simulink model "vfs_unity"  (R2022a)
settings: Solver=FixedStepAuto  StartTime=0.0  StopTime=inf  FixedStep=0.02  RelTol=1e-3
undefined symbols (not defined in the file): alpha, Angular, gd, Kc, Linear, ros_freq, Rx, Ry, Rz, T, var_max, X, Y, Z
libraries: simlib_vpc_coremath x35, robotlib x26, simlib_vpc_basic x14, simlib_vpc_gp x7, dspmtrx3 x5
(part 2 of 2)

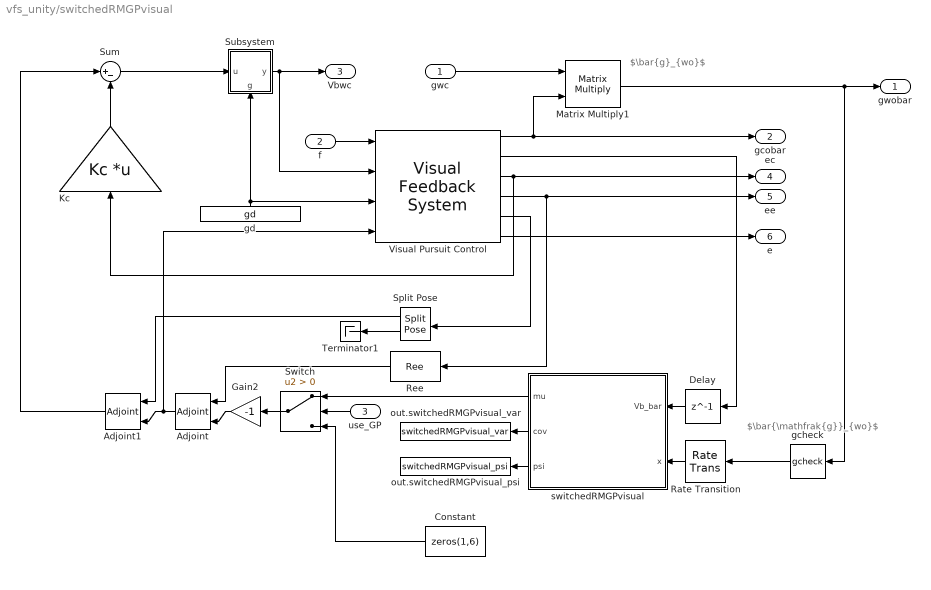
== system vfs_unity/switchedRMGPvisual ==
  note: $\bar{g}_{wo}$
  note: $\bar{\mathfrak{g}}_{wo}$
  gwc : Inport
  f : Inport  Port=2
  use_GP : Inport  Port=3
  Adjoint : simlib_vpc_basic/Adjoint  adjointtype=orientation
      settings: SourceProductName=VPC Library
  Adjoint1 : simlib_vpc_basic/Adjoint  adjointtype=orientation
      settings: SourceProductName=VPC Library
  Constant : Constant  Value=zeros(1,6)
  Delay : Delay  DelayLength=1
  Gain2 : Gain  Gain=-1
  Kc : Gain  Gain=Kc  Multiplication=Matrix(K*u) (u vector)
  Matrix Multiply1 : Product  Multiplication=Matrix(*)
  Rate Transition : RateTransition
  Ree : simlib_vpc_coremath/Ree
      settings: SourceProductName=VPC Library
  Split Pose : simlib_vpc_coremath/Split Pose  show_R=on  show_p=on
      settings: SourceProductName=VPC Library
  Subsystem : Subsystem
      settings: PortSchema="{\"entries\":[{\"content\":{\"sides\":[{\"content\":{\"connectorIds\":[\"In1\"]},\"type\":\"ConnectorPlacement.EquallySpacedRectSide\",\"uuid\":\"72e68008-5c4a-43a9-a560-64c6a31a0c08\"},{\"content\":{\"connectorIds\":[\"Out1\"],\"side\":\"RIGHT\"},\"type\":\"ConnectorPlacement.EquallySpacedRectSide\",\"uuid\":\"da07f5ff-2b2c-4c55-a2f2-34e133777503\"},{\"content\":{\"connectorIds\":[],\"side\":\"TOP\"},\"type\":\"ConnectorPlacement.EquallySpacedRectSide\",\"uuid\":\"6d174428-4364-4e89-aba7-4e9864808ab5\"},{\"content\":{\"connectorIds\":[\"In2\"],\"side\":\"BOTTOM\"},\"type\":\"ConnectorPlacement.EquallySpacedRectSide\",\"uuid\":\"f9633104-9c11-4d21-90a7-e0f886d9e92d\"},{\"content\":{\"connectorIds\":[],\"side\":\"HIDDEN\"},\"type\":\"ConnectorPlacement.EquallySpacedRectSide\",\"uuid\":\"662f08ae-9279-4a4f-85ea-81d97ead27d9\"}]},\"type\":\"ConnectorPlacement.EquallySpacedConnector\",\"uuid\":\"f3cd156c-cccd-47c6-b81c-6113f78efd58\"}],\"packageUris\":[\"http://schema.mathworks.com/mf0/Connector/R2020b\"],\"version\":\"1.0\"}"
      mask Display:
      | % Glitch in Matlab: If you define a line whose starting point and end point
      | % is equal, then the entire mask block is plotted in bold
      | plot([0,0],[0,0])
      | 
      | % Draw box
      | indent = 0.3;
      | ang=[0:0.2:pi/2, pi/2];
      | plot([0,1-indent],[0,0])
      | xp=indent*sin(ang)+1-indent;
      | yp=indent-indent*cos(ang);
      | plot(xp,yp);
      | plot([1,1,indent],[indent,1,1])
      | xp=indent-indent*sin(ang);
      | yp=1-indent+indent*cos(ang);
      | plot(xp,yp);
      | plot([0,0],[1-indent,0])
      | 
      | % Write label & ports
      | disp('-Ad_{(g_d)}','texmode','on')
      | text(0.5,0.2,'\fontsize{7}g_d','texmode','on')
  Sum : Sum  Inputs=|+-
  Switch : Switch  Criteria=u2 > Threshold  SaturateOnIntegerOverflow=off  InputSameDT=off
  Terminator1 : Terminator
  Visual Pursuit Control : simlib_vpc_basic/Visual Feedback System  gd_source=external  gd_value=[eye(4,3),ones(4,1)]  gcobar0=gco_init  Ke_source=internal  Ke=Ke  projection=on  camtype=Pinhole  fo=fp  lambda=lambda  show_Vbwo=on  show_ec=on  show_gce=on  show_ee=on  show_gee=off  show_e=on  show_nu=off  show_dgcobar=off  show_ue_aux=on
      settings: SourceProductName=VPC Library
  gcheck : simlib_vpc_coremath/gcheck
      settings: SourceProductName=VPC Library
  gd : Constant  Value=gd
  out.switchedRMGPvisual_psi : ToWorkspace  VariableName=switchedRMGPvisual_psi  SaveFormat=Structure With Time  SampleTime=-1
  out.switchedRMGPvisual_var : ToWorkspace  VariableName=switchedRMGPvisual_var  SaveFormat=Structure With Time  SampleTime=-1
  switchedRMGPvisual : Subsystem
      mask Display:
      | disp('Switched GP','texmode','on')
      | 
      | % Label ports
      | port_label('input',1,'V^b_{est}','texmode','on')
      | port_label('input',2,'x*','texmode','on')
      | port_label('output',1,'\mu','texmode','on')
      | port_label('output',2,'\Sigma','texmode','on')
      | port_label('output',3,'\psi_{est}','texmode','on')
  gwobar : Outport
  gcobar : Outport  Port=2
  Vbwc : Outport  Port=3
  ec : Outport  Port=4
  ee : Outport  Port=5
  e : Outport  Port=6
  wires:
  f/1 -> Visual Pursuit Control/1
  Matrix Multiply1/1 -> gwobar/1, gcheck/1
  Subsystem/1(y) -> Vbwc/1, Visual Pursuit Control/2
  gwc/1 -> Matrix Multiply1/1
  Visual Pursuit Control/5 -> Split Pose/1
  Kc/1 -> Sum/2
  Visual Pursuit Control/3 -> ec/1, Kc/1
  Visual Pursuit Control/4 -> Ree/1, ee/1
  gd/1 -> Subsystem/2(g), Visual Pursuit Control/3
  Visual Pursuit Control/1 -> Matrix Multiply1/2, gcobar/1
  Split Pose/1 -> Adjoint1/2
  Adjoint/1 -> Visual Pursuit Control/4, Adjoint1/1
  Ree/1 -> Adjoint/2
  Split Pose/2 -> Terminator1/1
  Gain2/1 -> Adjoint/1
  Sum/1 -> Subsystem/1(u)
  Adjoint1/1 -> Sum/1
  Visual Pursuit Control/6 -> e/1
  gcheck/1 -> Rate Transition/1
  switchedRMGPvisual/3(psi) -> out.switchedRMGPvisual_psi/1
  Rate Transition/1 -> switchedRMGPvisual/2(x)
  switchedRMGPvisual/2(cov) -> out.switchedRMGPvisual_var/1
  switchedRMGPvisual/1(mu) -> Switch/1
  Switch/1 -> Gain2/1
  Constant/1 -> Switch/3
  Delay/1 -> switchedRMGPvisual/1(Vb_bar)
  Visual Pursuit Control/2 -> Delay/1
  use_GP/1 -> Switch/2

== system vfs_unity/GP/Subsystem ==
  u : Inport
  g : Inport  Port=2
  Adjoint : simlib_vpc_basic/Adjoint  adjointtype=pose
      settings: SourceProductName=VPC Library
  Gain : Gain  Gain=-1
  y : Outport
  wires:
  Adjoint/1 -> y/1
  u/1 -> Gain/1
  g/1 -> Adjoint/2
  Gain/1 -> Adjoint/1

== system vfs_unity/Standard/Subsystem ==
  u : Inport
  g : Inport  Port=2
  Adjoint : simlib_vpc_basic/Adjoint  adjointtype=pose
      settings: SourceProductName=VPC Library
  Gain : Gain  Gain=-1
  y : Outport
  wires:
  Adjoint/1 -> y/1
  u/1 -> Gain/1
  g/1 -> Adjoint/2
  Gain/1 -> Adjoint/1

== system vfs_unity/switchedGP/Subsystem ==
  u : Inport
  g : Inport  Port=2
  Adjoint : simlib_vpc_basic/Adjoint  adjointtype=pose
      settings: SourceProductName=VPC Library
  Gain : Gain  Gain=-1
  y : Outport
  wires:
  Adjoint/1 -> y/1
  u/1 -> Gain/1
  g/1 -> Adjoint/2
  Gain/1 -> Adjoint/1

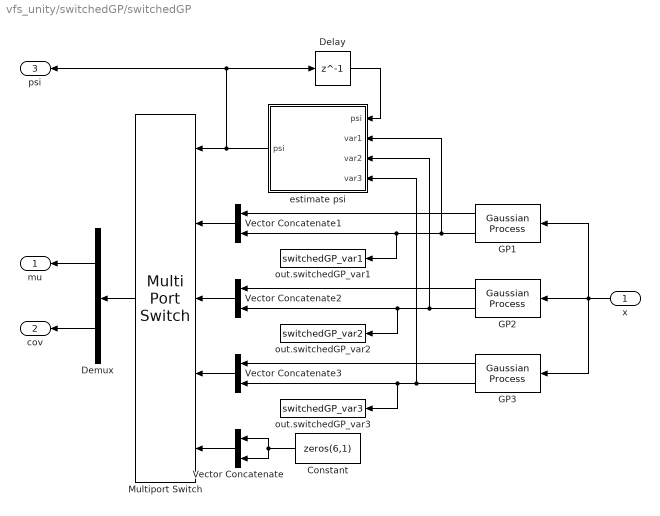
== system vfs_unity/switchedGP/switchedGP ==
  x : Inport
  Constant : Constant  Value=zeros(6,1)
  Delay : Delay  DelayLength=1
  Demux : Demux  Outputs=2
  GP1 : simlib_vpc_gp/Gaussian Process  X=X_switchedGP1  Y=Y_switchedGP1  sn=sn_switchedGP1  kernel=Squared Exponential ARD  hyp=hyp_switchedGP1  show_mean=on  show_variance=on  inv_fallback=off
      settings: SourceProductName=VPC Library
  GP2 : simlib_vpc_gp/Gaussian Process  X=X_switchedGP2  Y=Y_switchedGP2  sn=sn_switchedGP2  kernel=Squared Exponential ARD  hyp=hyp_switchedGP2  show_mean=on  show_variance=on  inv_fallback=off
      settings: SourceProductName=VPC Library
  GP3 : simlib_vpc_gp/Gaussian Process  X=X_switchedGP3  Y=Y_switchedGP3  sn=sn_switchedGP3  kernel=Squared Exponential ARD  hyp=hyp_switchedGP3  show_mean=on  show_variance=on  inv_fallback=off
      settings: SourceProductName=VPC Library
  Multiport Switch : MultiPortSwitch  DataPortForDefault=Additional data port  SaturateOnIntegerOverflow=off  InputSameDT=off
  Vector Concatenate{,1..3} (4 alike) : Concatenate
  estimate psi : MATLAB Function  TreatAsAtomicUnit=on
  out.switchedGP_var1 : ToWorkspace  VariableName=switchedGP_var1  SaveFormat=Structure With Time  SampleTime=-1
  out.switchedGP_var2 : ToWorkspace  VariableName=switchedGP_var2  SaveFormat=Structure With Time  SampleTime=-1
  out.switchedGP_var3 : ToWorkspace  VariableName=switchedGP_var3  SaveFormat=Structure With Time  SampleTime=-1
  mu : Outport
  cov : Outport  Port=2
  psi : Outport  Port=3
  wires:
  Constant/1 -> Vector Concatenate/2, Vector Concatenate/1
  Vector Concatenate/1 -> Multiport Switch/5
  Vector Concatenate1/1 -> Multiport Switch/2
  Multiport Switch/1 -> Demux/1
  Vector Concatenate2/1 -> Multiport Switch/3
  GP2/1 -> Vector Concatenate2/1
  GP1/1 -> Vector Concatenate1/1
  GP2/2 -> out.switchedGP_var2/1, Vector Concatenate2/2, estimate psi/3(var2)
  GP1/2 -> estimate psi/2(var1), out.switchedGP_var1/1, Vector Concatenate1/2
  Demux/1 -> mu/1
  Demux/2 -> cov/1
  estimate psi/1(psi) -> Multiport Switch/1, psi/1, Delay/1
  Delay/1 -> estimate psi/1("psi ")
  Vector Concatenate3/1 -> Multiport Switch/4
  GP3/1 -> Vector Concatenate3/1
  x/1 -> GP1/1, GP3/1, GP2/1
  GP3/2 -> estimate psi/4(var3), out.switchedGP_var3/1, Vector Concatenate3/2

== system vfs_unity/switchedRMGPvisual/Subsystem ==
  u : Inport
  g : Inport  Port=2
  Adjoint : simlib_vpc_basic/Adjoint  adjointtype=pose
      settings: SourceProductName=VPC Library
  Gain : Gain  Gain=-1
  y : Outport
  wires:
  Adjoint/1 -> y/1
  u/1 -> Gain/1
  g/1 -> Adjoint/2
  Gain/1 -> Adjoint/1

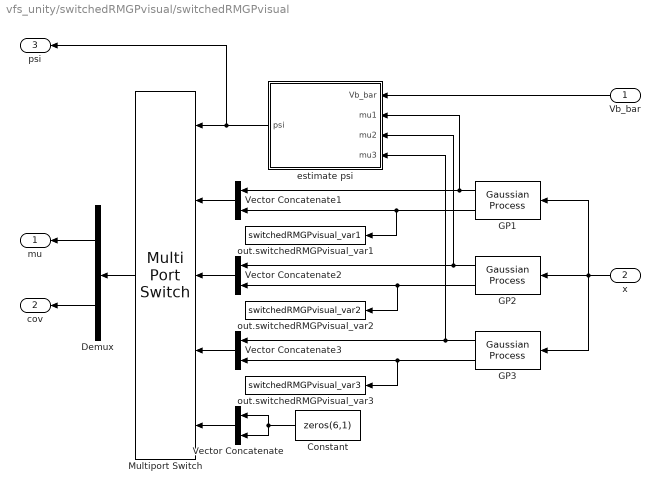
== system vfs_unity/switchedRMGPvisual/switchedRMGPvisual ==
  Vb_bar : Inport
  x : Inport  Port=2
  Constant : Constant  Value=zeros(6,1)
  Demux : Demux  Outputs=2
  GP1 : simlib_vpc_gp/Gaussian Process  X=X_switchedRMGPvisual1  Y=Y_switchedRMGPvisual1  sn=sn_switchedRMGPvisual1  kernel=SE3  hyp=hyp_switchedRMGPvisual1  show_mean=on  show_variance=on  inv_fallback=off
      settings: SourceProductName=VPC Library
  GP2 : simlib_vpc_gp/Gaussian Process  X=X_switchedRMGPvisual2  Y=Y_switchedRMGPvisual2  sn=sn_switchedRMGPvisual2  kernel=SE3  hyp=hyp_switchedRMGPvisual2  show_mean=on  show_variance=on  inv_fallback=off
      settings: SourceProductName=VPC Library
  GP3 : simlib_vpc_gp/Gaussian Process  X=X_switchedRMGPvisual3  Y=Y_switchedRMGPvisual3  sn=sn_switchedRMGPvisual3  kernel=SE3  hyp=hyp_switchedRMGPvisual3  show_mean=on  show_variance=on  inv_fallback=off
      settings: SourceProductName=VPC Library
  Multiport Switch : MultiPortSwitch  DataPortForDefault=Additional data port  SaturateOnIntegerOverflow=off  InputSameDT=off
  Vector Concatenate{,1..3} (4 alike) : Concatenate
  estimate psi : MATLAB Function  TreatAsAtomicUnit=on
  out.switchedRMGPvisual_var1 : ToWorkspace  VariableName=switchedRMGPvisual_var1  SaveFormat=Structure With Time  SampleTime=-1
  out.switchedRMGPvisual_var2 : ToWorkspace  VariableName=switchedRMGPvisual_var2  SaveFormat=Structure With Time  SampleTime=-1
  out.switchedRMGPvisual_var3 : ToWorkspace  VariableName=switchedRMGPvisual_var3  SaveFormat=Structure With Time  SampleTime=-1
  mu : Outport
  cov : Outport  Port=2
  psi : Outport  Port=3
  wires:
  Constant/1 -> Vector Concatenate/1, Vector Concatenate/2
  Vector Concatenate/1 -> Multiport Switch/5
  Vector Concatenate1/1 -> Multiport Switch/2
  Multiport Switch/1 -> Demux/1
  Vector Concatenate2/1 -> Multiport Switch/3
  GP2/1 -> estimate psi/3(mu2), Vector Concatenate2/1
  GP1/1 -> estimate psi/2(mu1), Vector Concatenate1/1
  GP2/2 -> out.switchedRMGPvisual_var2/1, Vector Concatenate2/2
  GP1/2 -> out.switchedRMGPvisual_var1/1, Vector Concatenate1/2
  Demux/1 -> mu/1
  Demux/2 -> cov/1
  estimate psi/1(psi) -> psi/1, Multiport Switch/1
  Vb_bar/1 -> estimate psi/1(Vb_bar)
  Vector Concatenate3/1 -> Multiport Switch/4
  x/1 -> GP1/1, GP3/1, GP2/1
  GP3/2 -> out.switchedRMGPvisual_var3/1, Vector Concatenate3/2
  GP3/1 -> estimate psi/4(mu3), Vector Concatenate3/1

== matlab function vfs_unity/Agent3 Cmd_vel/Convert Matlab To Unity ==
  data: vec_m input; vec_u output; rot input
function vec_u = matlab2unity(vec_m, rot) %#codegen
% Converts Matlab coordinate system to Unity system
%
% -----------
%
% Editor:
%   OMAINSKA Marco - Doctoral Student, Cybernetics
%       <marcoomainska@g.ecc.u-tokyo.ac.jp>
% Property of: Fujita-Yamauchi Lab, The University of Tokyo, 2022
% Website: https://www.scl.ipc.i.u-tokyo.ac.jp

%------------- BEGIN CODE --------------
vec_m = vec_m(:);

% define output dimension
vec_u = zeros(size(vec_m));

% apply rot-transform if given
vec_m = adjoint(rot,'orientation') * vec_m;

% transform to unity system
vec_u(1) = vec_m(1);
vec_u(2) = vec_m(3);
vec_u(3) = vec_m(2);
vec_u(4) = -vec_m(4);
vec_u(5) = -vec_m(6);
vec_u(6) = -vec_m(5);

%------------- END CODE --------------
end

== matlab function vfs_unity/Set Target Estimate3/Convert Matlab To Unity ==
  data: vec_m input; vec_u output; rot input
function vec_u = matlab2unity(vec_m, rot) %#codegen
% Converts Matlab coordinate system to Unity system
%
% -----------
%
% Editor:
%   OMAINSKA Marco - Doctoral Student, Cybernetics
%       <marcoomainska@g.ecc.u-tokyo.ac.jp>
% Property of: Fujita-Yamauchi Lab, The University of Tokyo, 2022
% Website: https://www.scl.ipc.i.u-tokyo.ac.jp

%------------- BEGIN CODE --------------
vec_m = vec_m(:);

% define output dimension
vec_u = zeros(size(vec_m));

% apply rot-transform if given
vec_m = adjoint(rot,'orientation') * vec_m;

% transform to unity system
vec_u(1) = vec_m(1);
vec_u(2) = vec_m(3);
vec_u(3) = vec_m(2);
vec_u(4) = -vec_m(4);
vec_u(5) = -vec_m(6);
vec_u(6) = -vec_m(5);

%------------- END CODE --------------
end

== matlab function vfs_unity/Agent4 Cmd_vel/Convert Matlab To Unity ==
  data: vec_m input; vec_u output; rot input
function vec_u = matlab2unity(vec_m, rot) %#codegen
% Converts Matlab coordinate system to Unity system
%
% -----------
%
% Editor:
%   OMAINSKA Marco - Doctoral Student, Cybernetics
%       <marcoomainska@g.ecc.u-tokyo.ac.jp>
% Property of: Fujita-Yamauchi Lab, The University of Tokyo, 2022
% Website: https://www.scl.ipc.i.u-tokyo.ac.jp

%------------- BEGIN CODE --------------
vec_m = vec_m(:);

% define output dimension
vec_u = zeros(size(vec_m));

% apply rot-transform if given
vec_m = adjoint(rot,'orientation') * vec_m;

% transform to unity system
vec_u(1) = vec_m(1);
vec_u(2) = vec_m(3);
vec_u(3) = vec_m(2);
vec_u(4) = -vec_m(4);
vec_u(5) = -vec_m(6);
vec_u(6) = -vec_m(5);

%------------- END CODE --------------
end

== matlab function vfs_unity/Set Target Estimate4/Convert Matlab To Unity ==
  data: vec_m input; vec_u output; rot input
function vec_u = matlab2unity(vec_m, rot) %#codegen
% Converts Matlab coordinate system to Unity system
%
% -----------
%
% Editor:
%   OMAINSKA Marco - Doctoral Student, Cybernetics
%       <marcoomainska@g.ecc.u-tokyo.ac.jp>
% Property of: Fujita-Yamauchi Lab, The University of Tokyo, 2022
% Website: https://www.scl.ipc.i.u-tokyo.ac.jp

%------------- BEGIN CODE --------------
vec_m = vec_m(:);

% define output dimension
vec_u = zeros(size(vec_m));

% apply rot-transform if given
vec_m = adjoint(rot,'orientation') * vec_m;

% transform to unity system
vec_u(1) = vec_m(1);
vec_u(2) = vec_m(3);
vec_u(3) = vec_m(2);
vec_u(4) = -vec_m(4);
vec_u(5) = -vec_m(6);
vec_u(6) = -vec_m(5);

%------------- END CODE --------------
end

== matlab function vfs_unity/Agent4 Pose gwc/Convert Unity To Matlab ==
  data: vec_u input; vec_m output; rot input
function vec_m = unity2matlab(vec_u, rot) %#codegen
% Converts Unity coordinate system to Matlab system
%
% -----------
%
% Editor:
%   OMAINSKA Marco - Doctoral Student, Cybernetics
%       <marcoomainska@g.ecc.u-tokyo.ac.jp>
% Property of: Fujita-Yamauchi Lab, The University of Tokyo, 2022
% Website: https://www.scl.ipc.i.u-tokyo.ac.jp

%------------- BEGIN CODE --------------
vec_u = vec_u(:);

% define output dimension
vec_m = zeros(size(vec_u));

% transform to unity system
vec_m(1) = vec_u(1);
vec_m(2) = vec_u(3);
vec_m(3) = vec_u(2);
vec_m(4) = -vec_u(4);
vec_m(5) = -vec_u(6);
vec_m(6) = -vec_u(5);

% apply rot-transform if given
vec_m = adjoint(rot,'orientation') * vec_m;

%------------- END CODE --------------
end

== matlab function vfs_unity/switchedGP/switchedGP/estimate psi ==
  data: psi input; var1 input; psi output; var2 input; var3 input; var_max parameter; T parameter; alpha parameter
function psi = estim_psi(psi,var1,var2,var3,var_max,T,alpha)
%%ESTIM_PSI estimates the switching signal s(t)
%
% Editor:
%   OMAINSKA Marco - Doctoral Student, Cybernetics
%       <marcoomainska@g.ecc.u-tokyo.ac.jp>
% Review:
%   YAMAUCHI Junya - Assistant Professor
%       <junya_yamauchi@ipc.i.u-tokyo.ac.jp>
%
% Property of: Fujita-Yamauchi Lab, University of Tokyo, 2021
% e-mail: marcoomainska@g.ecc.u-tokyo.ac.jp
% Website: https://www.scl.ipc.i.u-tokyo.ac.jp
% February 2022
%
%------------- BEGIN CODE --------------

% calculate norms
var_norm = zeros(3,1);
% disp(var1);
var_norm(1) = norm(dot(alpha,sqrt(var1)),2)/var_max(1);
var_norm(2) = norm(dot(alpha,sqrt(var2)),2)/var_max(2);
var_norm(3) = norm(dot(alpha,sqrt(var3)),2)/var_max(3);

% estimate switching
if psi == 0 % init case: psi is zero
    [~,psi] = min(var_norm); % find the smallest ||var||/var_max
else
    [~,psi_new] = min(var_norm); % find the smallest ||var||/var_max
    if var_norm(psi) > var_norm(psi_new) + T
        psi = psi_new;
    end
end

% fail safe case
if isnan(psi)
    psi = 0;
end

%-------------- END CODE ---------------
end

== matlab function vfs_unity/Agent1 Cmd_vel/Convert Matlab To Unity ==
  data: vec_m input; vec_u output; rot input
function vec_u = matlab2unity(vec_m, rot) %#codegen
% Converts Matlab coordinate system to Unity system
%
% -----------
%
% Editor:
%   OMAINSKA Marco - Doctoral Student, Cybernetics
%       <marcoomainska@g.ecc.u-tokyo.ac.jp>
% Property of: Fujita-Yamauchi Lab, The University of Tokyo, 2022
% Website: https://www.scl.ipc.i.u-tokyo.ac.jp

%------------- BEGIN CODE --------------
vec_m = vec_m(:);

% define output dimension
vec_u = zeros(size(vec_m));

% apply rot-transform if given
vec_m = adjoint(rot,'orientation') * vec_m;

% transform to unity system
vec_u(1) = vec_m(1);
vec_u(2) = vec_m(3);
vec_u(3) = vec_m(2);
vec_u(4) = -vec_m(4);
vec_u(5) = -vec_m(6);
vec_u(6) = -vec_m(5);

%------------- END CODE --------------
end

== matlab function vfs_unity/Agent1 Pose gwc/Convert Unity To Matlab ==
  data: vec_u input; vec_m output; rot input
function vec_m = unity2matlab(vec_u, rot) %#codegen
% Converts Unity coordinate system to Matlab system
%
% -----------
%
% Editor:
%   OMAINSKA Marco - Doctoral Student, Cybernetics
%       <marcoomainska@g.ecc.u-tokyo.ac.jp>
% Property of: Fujita-Yamauchi Lab, The University of Tokyo, 2022
% Website: https://www.scl.ipc.i.u-tokyo.ac.jp

%------------- BEGIN CODE --------------
vec_u = vec_u(:);

% define output dimension
vec_m = zeros(size(vec_u));

% transform to unity system
vec_m(1) = vec_u(1);
vec_m(2) = vec_u(3);
vec_m(3) = vec_u(2);
vec_m(4) = -vec_u(4);
vec_m(5) = -vec_u(6);
vec_m(6) = -vec_u(5);

% apply rot-transform if given
vec_m = adjoint(rot,'orientation') * vec_m;

%------------- END CODE --------------
end

== matlab function vfs_unity/Set Target Estimate1/Convert Matlab To Unity ==
  data: vec_m input; vec_u output; rot input
function vec_u = matlab2unity(vec_m, rot) %#codegen
% Converts Matlab coordinate system to Unity system
%
% -----------
%
% Editor:
%   OMAINSKA Marco - Doctoral Student, Cybernetics
%       <marcoomainska@g.ecc.u-tokyo.ac.jp>
% Property of: Fujita-Yamauchi Lab, The University of Tokyo, 2022
% Website: https://www.scl.ipc.i.u-tokyo.ac.jp

%------------- BEGIN CODE --------------
vec_m = vec_m(:);

% define output dimension
vec_u = zeros(size(vec_m));

% apply rot-transform if given
vec_m = adjoint(rot,'orientation') * vec_m;

% transform to unity system
vec_u(1) = vec_m(1);
vec_u(2) = vec_m(3);
vec_u(3) = vec_m(2);
vec_u(4) = -vec_m(4);
vec_u(5) = -vec_m(6);
vec_u(6) = -vec_m(5);

%------------- END CODE --------------
end

== matlab function vfs_unity/switchedRMGPvisual/switchedRMGPvisual/estimate psi ==
  data: Vb_bar input; mu1 input; psi output; mu2 input; mu3 input
function psi = estim_psi(Vb_bar,mu1,mu2,mu3)
%%ESTIM_PSI estimates the switching signal s(t)
%
% Editor:
%   OMAINSKA Marco - Doctoral Student, Cybernetics
%       <marcoomainska@g.ecc.u-tokyo.ac.jp>
% Review:
%   YAMAUCHI Junya - Assistant Professor
%       <junya_yamauchi@ipc.i.u-tokyo.ac.jp>
%
% Property of: Fujita-Yamauchi Lab, University of Tokyo, 2021
% e-mail: marcoomainska@g.ecc.u-tokyo.ac.jp
% Website: https://www.scl.ipc.i.u-tokyo.ac.jp
% February 2022
%
%------------- BEGIN CODE --------------

Vbee_vec = zeros(1,3);
Vbee_vec(1) = norm(Vb_bar-mu1,2);
Vbee_vec(2) = norm(Vb_bar-mu2,2);
Vbee_vec(3) = norm(Vb_bar-mu3,2);

[~,psi] = min(Vbee_vec);

%-------------- END CODE ---------------
end

== matlab function vfs_unity/Target Pose gwo/Convert Unity To Matlab ==
  data: vec_u input; vec_m output; rot input
function vec_m = unity2matlab(vec_u, rot) %#codegen
% Converts Unity coordinate system to Matlab system
%
% -----------
%
% Editor:
%   OMAINSKA Marco - Doctoral Student, Cybernetics
%       <marcoomainska@g.ecc.u-tokyo.ac.jp>
% Property of: Fujita-Yamauchi Lab, The University of Tokyo, 2022
% Website: https://www.scl.ipc.i.u-tokyo.ac.jp

%------------- BEGIN CODE --------------
vec_u = vec_u(:);

% define output dimension
vec_m = zeros(size(vec_u));

% transform to unity system
vec_m(1) = vec_u(1);
vec_m(2) = vec_u(3);
vec_m(3) = vec_u(2);
vec_m(4) = -vec_u(4);
vec_m(5) = -vec_u(6);
vec_m(6) = -vec_u(5);

% apply rot-transform if given
vec_m = adjoint(rot,'orientation') * vec_m;

%------------- END CODE --------------
end

== matlab function vfs_unity/Agent2 Pose gwc/Convert Unity To Matlab ==
  data: vec_u input; vec_m output; rot input
function vec_m = unity2matlab(vec_u, rot) %#codegen
% Converts Unity coordinate system to Matlab system
%
% -----------
%
% Editor:
%   OMAINSKA Marco - Doctoral Student, Cybernetics
%       <marcoomainska@g.ecc.u-tokyo.ac.jp>
% Property of: Fujita-Yamauchi Lab, The University of Tokyo, 2022
% Website: https://www.scl.ipc.i.u-tokyo.ac.jp

%------------- BEGIN CODE --------------
vec_u = vec_u(:);

% define output dimension
vec_m = zeros(size(vec_u));

% transform to unity system
vec_m(1) = vec_u(1);
vec_m(2) = vec_u(3);
vec_m(3) = vec_u(2);
vec_m(4) = -vec_u(4);
vec_m(5) = -vec_u(6);
vec_m(6) = -vec_u(5);

% apply rot-transform if given
vec_m = adjoint(rot,'orientation') * vec_m;

%------------- END CODE --------------
end

== matlab function vfs_unity/Agent3 Pose gwc/Convert Unity To Matlab ==
  data: vec_u input; vec_m output; rot input
function vec_m = unity2matlab(vec_u, rot) %#codegen
% Converts Unity coordinate system to Matlab system
%
% -----------
%
% Editor:
%   OMAINSKA Marco - Doctoral Student, Cybernetics
%       <marcoomainska@g.ecc.u-tokyo.ac.jp>
% Property of: Fujita-Yamauchi Lab, The University of Tokyo, 2022
% Website: https://www.scl.ipc.i.u-tokyo.ac.jp

%------------- BEGIN CODE --------------
vec_u = vec_u(:);

% define output dimension
vec_m = zeros(size(vec_u));

% transform to unity system
vec_m(1) = vec_u(1);
vec_m(2) = vec_u(3);
vec_m(3) = vec_u(2);
vec_m(4) = -vec_u(4);
vec_m(5) = -vec_u(6);
vec_m(6) = -vec_u(5);

% apply rot-transform if given
vec_m = adjoint(rot,'orientation') * vec_m;

%------------- END CODE --------------
end

== matlab function vfs_unity/Agent2 Cmd_vel/Convert Matlab To Unity ==
  data: vec_m input; vec_u output; rot input
function vec_u = matlab2unity(vec_m, rot) %#codegen
% Converts Matlab coordinate system to Unity system
%
% -----------
%
% Editor:
%   OMAINSKA Marco - Doctoral Student, Cybernetics
%       <marcoomainska@g.ecc.u-tokyo.ac.jp>
% Property of: Fujita-Yamauchi Lab, The University of Tokyo, 2022
% Website: https://www.scl.ipc.i.u-tokyo.ac.jp

%------------- BEGIN CODE --------------
vec_m = vec_m(:);

% define output dimension
vec_u = zeros(size(vec_m));

% apply rot-transform if given
vec_m = adjoint(rot,'orientation') * vec_m;

% transform to unity system
vec_u(1) = vec_m(1);
vec_u(2) = vec_m(3);
vec_u(3) = vec_m(2);
vec_u(4) = -vec_m(4);
vec_u(5) = -vec_m(6);
vec_u(6) = -vec_m(5);

%------------- END CODE --------------
end

== matlab function vfs_unity/Set Target Estimate2/Convert Matlab To Unity ==
  data: vec_m input; vec_u output; rot input
function vec_u = matlab2unity(vec_m, rot) %#codegen
% Converts Matlab coordinate system to Unity system
%
% -----------
%
% Editor:
%   OMAINSKA Marco - Doctoral Student, Cybernetics
%       <marcoomainska@g.ecc.u-tokyo.ac.jp>
% Property of: Fujita-Yamauchi Lab, The University of Tokyo, 2022
% Website: https://www.scl.ipc.i.u-tokyo.ac.jp

%------------- BEGIN CODE --------------
vec_m = vec_m(:);

% define output dimension
vec_u = zeros(size(vec_m));

% apply rot-transform if given
vec_m = adjoint(rot,'orientation') * vec_m;

% transform to unity system
vec_u(1) = vec_m(1);
vec_u(2) = vec_m(3);
vec_u(3) = vec_m(2);
vec_u(4) = -vec_m(4);
vec_u(5) = -vec_m(6);
vec_u(6) = -vec_m(5);

%------------- END CODE --------------
end
